simulink model "ndu"  (R2021a)
settings: Solver=VariableStepAuto  StartTime=0.0  StopTime=250  RelTol=1e-3
model workspace (MAT data in the model file):
  J1 = 0.1
  K1 = 0.1
  K2 = 0.0015625
settings Model: Creator=Jurica Vučković  LastModifiedBy=Jurica Vučković
settings DataIOCC: ExternalInput=ts  LoadExternalInput=on  OutputSaveName=w2

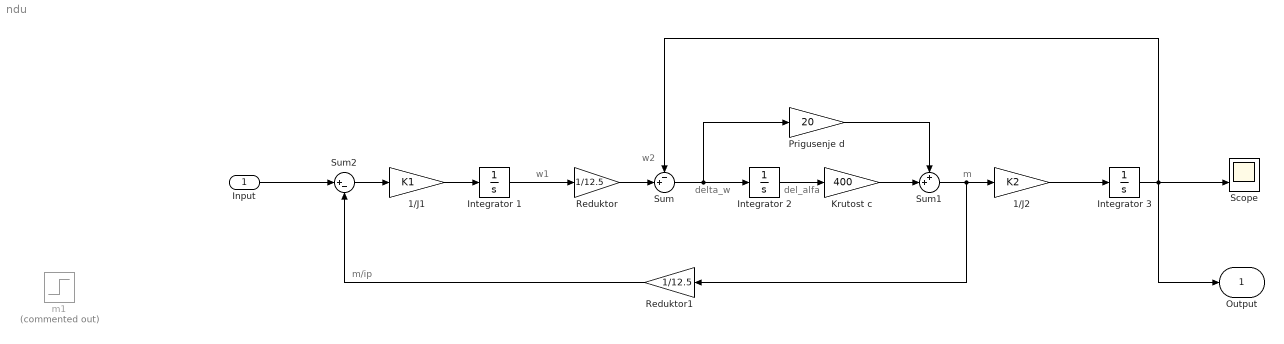
== system ndu ==
  note: m/ip
  note: m
  note: del_alfa
  note: w2
  note: delta_w
  note: w1
  Input : Inport
  1/J1 : Gain  Gain=K1
  1/J2 : Gain  Gain=K2
  Integrator 1 : Integrator
  Integrator 2 : Integrator  UpperSaturationLimit=0.2  LowerSaturationLimit=-0.2
  Integrator 3 : Integrator
  Krutost c : Gain  Gain=400
  Prigusenje d : Gain  Gain=20
  Reduktor : Gain  Gain=1/12.5
  Reduktor1 : Gain  Gain=1/12.5
  Scope : Scope  NumInputPorts=2
  Sum : Sum  Inputs=-+|
  Sum1 : Sum  Inputs=++|
  Sum2 : Sum  Inputs=|+-
  m1 : Step  Commented=on  After=20  SampleTime=0
  Output : Outport  SignalName=w2
  wires:
  1/J1/1 -> Integrator 1/1
  Integrator 1/1 -> Reduktor/1
  Reduktor/1 -> Sum/2
  Krutost c/1 -> Sum1/2
  Sum/1 -> Prigusenje d/1, Integrator 2/1
  Prigusenje d/1 -> Sum1/1
  1/J2/1 -> Integrator 3/1
  Integrator 3/1 -> Output/1, Scope/2, Sum/1
  Sum2/1 -> 1/J1/1
  Sum1/1 -> Reduktor1/1, 1/J2/1
  Reduktor1/1 -> Sum2/2
  Input/1 -> Sum2/1
  Integrator 2/1 -> Krutost c/1
